simulink model "simu"  (R2023a)
settings: Solver=VariableStepAuto  StartTime=0.0  StopTime=10.0  RelTol=1e-3
settings Model: Creator=MTS  LastModifiedBy=MTS

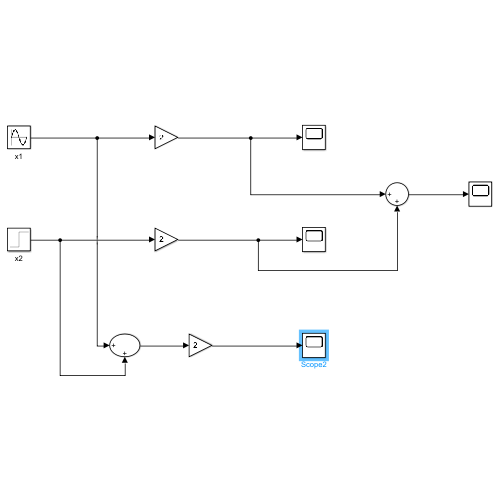
[thumbnail: Simulink's stored preview of the top-level diagram]
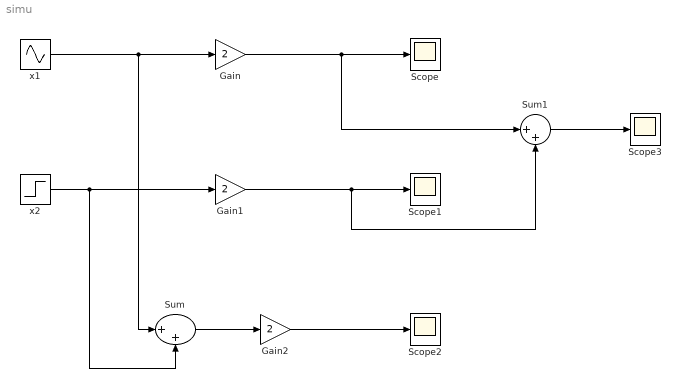
== system simu ==
  Gain : Gain  Gain=2
  Gain1 : Gain  Gain=2
  Gain2 : Gain  Gain=2
  Scope{,1..3} (4 alike) : Scope
  Sum : Sum  Inputs=|++
  Sum1 : Sum  Inputs=|++
  x1 : Sin  SampleTime=0
  x2 : Step  SampleTime=0
  wires:
  x2/1 -> Sum/2, Gain1/1
  Gain/1 -> Sum1/1, Scope/1
  Gain1/1 -> Sum1/2, Scope1/1
  x1/1 -> Gain/1, Sum/1
  Sum/1 -> Gain2/1
  Gain2/1 -> Scope2/1
  Sum1/1 -> Scope3/1
